simulink library "ControLibrary"  (R2015b)
settings: Solver=ode45  SolverMode=SingleTasking  StartTime=0.0  StopTime=10.0  RelTol=1e-3
values from neighbouring files (symbols this model uses):
  ControlSampleTime = 1/8000    (= 0.000125)    [initTPHardware.m]
  DCCC = initDCCC(LCL,SM)    [Sim_TP3_VSM_init.m]    (also in initDCCC.m = initHSS(LCL,SM))
undefined symbols (not defined in the file or in its folder): CCCTRL, DiscIntNeverNeededParam, VSMCTRL
undefined symbols (not defined in the file): HSS, VSMCC
libraries: FriedrichLibrary x46, simulink x23, simulink_extras x4, ControLibrary x2, ctrl_basic x2
(part 1 of 4)
settings Model: Creator=fwelck  LastModifiedBy=fwelck
settings DataIOCC: SaveFormat=Array
settings OptimizationCC: BlockReduction=off  BooleanDataType=off
settings DebuggingCC: SaveWithParameterizedLinksMsg=none  UnderspecifiedInitializationDetection=Classic  MergeDetectMultiDrivingBlocksExec=none  SignalResolutionControl=TryResolveAllWithWarning  StrictBusMsg=Warning
settings HardwareCC: ProdBitPerPointer=32  ProdLargestAtomicFloat=None  ProdIntDivRoundTo=Undefined  ProdEndianess=Unspecified  ProdWordSize=32  ProdHWDeviceType=32-bit Generic  TargetUnknown=on
settings GRTTargetCC: GeneratePreprocessorConditionals=Disable all
settings ConfigComp: CovModelRefEnable=Off  CovSFcnEnable=off

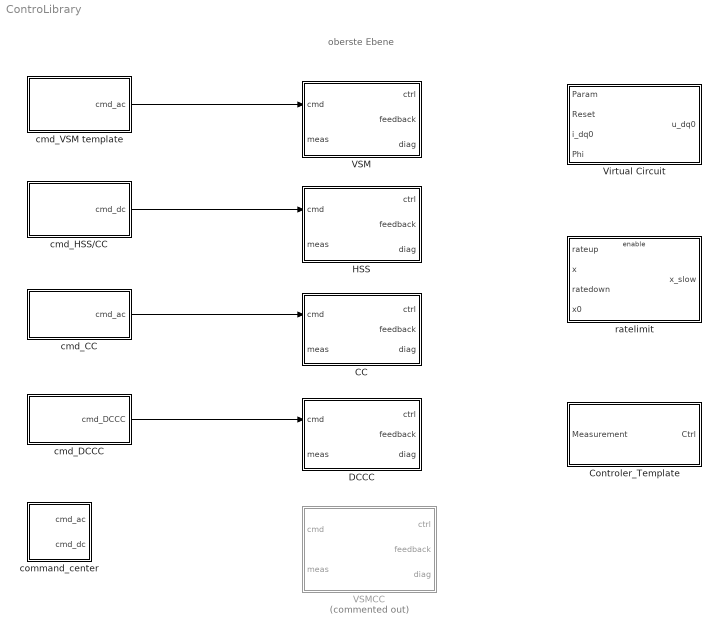
== system ControLibrary ==
  note: oberste Ebene
  CC : Subsystem  InitFcn=createTriphaseBus  mask{Ctrl=CCCTRL, pu=CCCTRL.PU, DoN=off}
      mask prompts: Ctrl "Param Struct"; pu "PU-System"; DoN "N Leiter Schalten (4 Phasen)"
      mask init:
      | if DoN
      |     NrChannels=4;
      | else
      |     NrChannels=3;
      | end
  Controler_Template : Subsystem
  DCCC : Subsystem  InitFcn=createTriphaseBus  mask{Ctrl=DCCC, PU=DCCC.PU}
      mask prompts: Ctrl "ParamStruct"; PU "PU-System"
      mask init:
      | NrChannels = 3;
  HSS : Subsystem  InitFcn=createTriphaseBus  mask{Ctrl=HSS, PU=VSMCTRL.PU}
      mask prompts: Ctrl "ParamStruct"; PU "PU-System"
  VSM : Subsystem  ClipboardFcn=createTriphaseBus  mask{Ctrl=VSMCTRL, pu=VSMCTRL.PU, DoN=off}
      mask prompts: Ctrl "ParamStruct"; pu "PU-System"; DoN "N Leiter Schalten (4 Phasen)"
      mask init:
      | if DoN
      |     NrChannels=4;
      | else
      |     NrChannels=3;
      | end
  VSMCC : Subsystem  Commented=on  mask{Ctrl=VSMCC, DoN=off}
      mask prompts: Ctrl "ParamStruct"; DoN "N Leiter Schalten (4 Phasen)"
      mask init:
      | if DoN
      |     NrChannels=4;
      | else
      |     NrChannels=3;
      | end
  Virtual Circuit : Subsystem
  cmd_CC : Subsystem
  cmd_DCCC : Subsystem
  cmd_HSS/CC : Subsystem
  cmd_VSM template : Subsystem
  command_center : Subsystem
  ratelimit : Subsystem  mask{Ts=ControlSampleTime}
      mask DialogControl ParameterGroupVar Prompt: Rate Limiter
  wires:
  cmd_VSM template/1(cmd_ac) -> VSM/1(cmd)
  cmd_HSS/CC/1(cmd_dc) -> HSS/1(cmd)
  cmd_CC/1(cmd_ac) -> CC/1(cmd)
  cmd_DCCC/1(cmd_DCCC) -> DCCC/1(cmd)

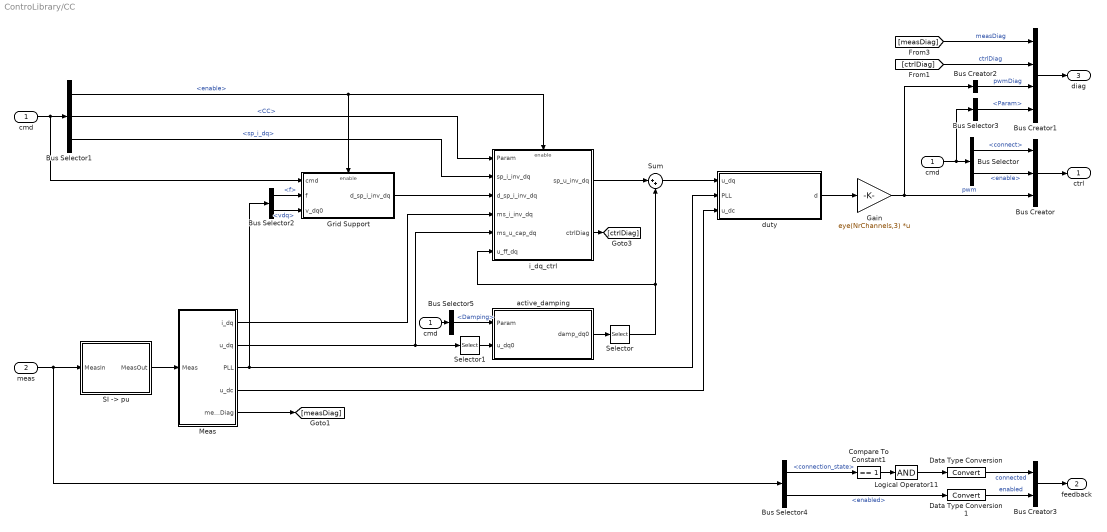
== system ControLibrary/CC ==
  cmd : Inport
  meas : Inport  Port=2
  "  cmd  " : InportShadow
  Bus Creator : BusCreator  Inputs=3
  Bus Creator1 : BusCreator  Inputs=4
  Bus Creator2 : BusCreator  Inputs=1
  Bus Selector : BusSelector  OutputSignals=Manage.connect,Manage.enable
  Bus Selector1 : BusSelector  OutputSignals=Manage.enable,Param.CC,sp_i_dq
  Bus Selector2 : BusSelector  OutputSignals=f,vdq
  Bus Selector3 : BusSelector  OutputSignals=Param
  Bus Selector4 : BusSelector  OutputSignals=connection_state,enabled
  Bus Selector5 : BusSelector  OutputSignals=Damping
  Bus Creator3 : BusCreator  Inputs=2  OutDataTypeStr=Bus: FeedbackACBus
  Compare To Constant1 : simulink/Logic and Bit Operations/Compare To Constant  relop===  const=1  OutDataTypeStr=boolean
  Data Type Conversion : DataTypeConversion
  Data Type Conversion1 : DataTypeConversion
  Gain : Gain  Gain=eye(NrChannels,3)  Multiplication=Matrix(K*u)
  Grid Support : Subsystem  mask{Omegab=pu.omegab, tauhf=1e-3}
      mask DialogControl dfdtRegler Prompt: df/dt Regler
  Logical Operator11 : Logic  Inputs=1  AllPortsSameDT=off  OutDataTypeStr=boolean
  Meas : Subsystem  mask{PLL=Ctrl.PLL}
      mask prompts: PLL "PLL Parameter"
  "SI -> pu" : Subsystem  mask{PU=pu}
      mask prompts: PU "PU System"
      mask DialogControl ParameterGroupVar Prompt: Per Unit
  Selector : Selector  InputPortWidth=3  IndexOptions=Index vector (dialog)  Indices=[1 2]  OutputSizes=1
  Selector1 : Selector  InputPortWidth=2  IndexOptions=Index vector (dialog)  Indices=[1 2 2]  OutputSizes=1
  Sum : Sum  Inputs=|++
  active_damping : Subsystem
  "cmd " : InportShadow
  duty : Subsystem
  i_dq_ctrl : Subsystem
  ctrl : Outport
  feedback : Outport  Port=2
  diag : Outport  Port=3
  wires:
  Selector1/1 -> active_damping/2(u_dq0)
  Selector/1 -> Sum/2, i_dq_ctrl/6(u_ff_dq)
  Bus Selector5/1 -> active_damping/1(Param)  "<Damping>"
  "  cmd  "/1 -> Bus Selector5/1
  Sum/1 -> duty/1(u_dq)
  i_dq_ctrl/1(sp_u_inv_dq) -> Sum/1
  Bus Selector1/2 -> i_dq_ctrl/1(Param)  "<CC>"
  Logical Operator11/1 -> Data Type Conversion/1
  Bus Selector4/1 -> Compare To Constant1/1  "<connection_state>"
  Compare To Constant1/1 -> Logical Operator11/1
  Bus Selector4/2 -> Data Type Conversion1/1  "<enabled>"
  Data Type Conversion1/1 -> Bus Creator3/2  "enabled"
  Bus Creator3/1 -> feedback/1
  Data Type Conversion/1 -> Bus Creator3/1  "connected"
  Bus Creator2/1 -> Bus Creator1/3  "pwmDiag"
  Bus Selector3/1 -> Bus Creator1/4  "<Param>"
  cmd/1 -> Bus Selector/1, Bus Selector3/1
  Grid Support/1(d_sp_i_inv_dq) -> i_dq_ctrl/3(d_sp_i_inv_dq)
  Bus Selector1/3 -> i_dq_ctrl/2(sp_i_inv_dq)  "<sp_i_dq>"
  Bus Selector1/1 -> Grid Support/Enable, i_dq_ctrl/Enable  "<enable>"
  "cmd "/1 -> Grid Support/1(cmd), Bus Selector1/1
  Bus Selector2/1 -> Grid Support/2(f)  "<f>"
  active_damping/1(damp_dq0) -> Selector/1
  Bus Creator1/1 -> diag/1
  [ctrlDiag] -> Bus Creator1/2  "ctrlDiag"
  [measDiag] -> Bus Creator1/1  "measDiag"
  Meas/5(measDiag) -> [measDiag]
  i_dq_ctrl/2(ctrlDiag) -> [ctrlDiag]
  duty/1(d) -> Gain/1
  Meas/4(u_dc) -> duty/3(u_dc)
  Meas/3(PLL) -> duty/2(PLL), Bus Selector2/1
  Meas/2(u_dq) -> i_dq_ctrl/5(ms_u_cap_dq), Selector1/1
  Gain/1 -> Bus Creator/3, Bus Creator2/1  "pwm"
  Meas/1(i_dq) -> i_dq_ctrl/4(ms_i_inv_dq)
  Bus Selector/2 -> Bus Creator/2  "<enable>"
  Bus Creator/1 -> ctrl/1
  Bus Selector/1 -> Bus Creator/1  "<connect>"
  meas/1 -> Bus Selector4/1, "SI -> pu"/1(MeasIn)
  "SI -> pu"/1(MeasOut) -> Meas/1(Meas)
  Bus Selector2/2 -> Grid Support/3(v_dq0)  "<vdq>"

== system ControLibrary/Controler_Template ==
  Measurement : Inport
  Bus Creator : BusCreator  Inputs=3
  Bus Selector : BusSelector  OutputSignals=Inv1,Inv2
  Constant : Constant  Value=0
  Constant1 : Constant  Value=0
  INV1_ctrl : Subsystem
  INV2_ctrl : Subsystem
  preload : Step  Time=0.1  SampleTime=0
  Ctrl : Outport
  wires:
  Bus Selector/2 -> INV2_ctrl/2(meas)  "<Inv2>"
  Bus Selector/1 -> INV1_ctrl/2(meas)  "<Inv1>"
  Measurement/1 -> Bus Selector/1
  preload/1 -> Bus Creator/1  "preload"
  Bus Creator/1 -> Ctrl/1
  INV2_ctrl/1(ctrl) -> Bus Creator/3  "Inv2"
  INV1_ctrl/1(ctrl) -> Bus Creator/2  "Inv1"
  Constant1/1 -> INV1_ctrl/1(cmd)
  Constant/1 -> INV2_ctrl/1(cmd)

== system ControLibrary/DCCC ==
  cmd : Inport
  meas : Inport  Port=2
  BUS_GENERATION : Subsystem
  CONTROL : Subsystem
  MANAGEMENT : Subsystem  mask{UDCbusSpMax=Ctrl.Mgn.UDCbusSpMax, UDCbusSpMin=Ctrl.Mgn.UDCbusSpMin, UDCbusSpRateUp=Ctrl.Mgn.UDCbusSpRateUp, UDCbusSpRateDown=Ctrl.Mgn.UDCbusSpRateDown, PU=PU}
      mask prompts: UDCbusSpMax "UDCbusSpMax [V]"; UDCbusSpMin "UDCbusSpMin [V]"; UDCbusSpRateUp "UDCbusSpRateUp [V/s]"; UDCbusSpRateDown "UDCbusSpRateDown [V/s]"; PU "PU-System"
      mask DialogControl GrpHssMgn Prompt: HSS Management
  Meas : Subsystem  mask(Messeinrichtung für VSM mit CC){PU=PU, PLL=Ctrl.PLL}
      mask prompts: PU "PU System"; PLL "PLL Parameters"
      mask help:
      | PU System(.Vb, .Ib)
      |
      | PLL Parameter (.kp, .ki)
      |
      | Parameter nicht auf der Maske:
      | NrChannels
      | ControlSampleTime
  ctrl : Outport  LockScale=on
  feedback : Outport  Port=2
  diag : Outport  Port=3
  wires:
  meas/1 -> Meas/1(MEASIN)
  Meas/1(MEAS) -> MANAGEMENT/2(MEAS), CONTROL/2(MEAS)
  cmd/1 -> MANAGEMENT/1(CMD)
  MANAGEMENT/1(MANAGE) -> CONTROL/1(MANAGE), BUS_GENERATION/1(MANAGE)
  CONTROL/2(diagCtrl) -> diag/1
  CONTROL/1(CONTROL) -> BUS_GENERATION/2(CONTROL)
  BUS_GENERATION/1(ctrl) -> ctrl/1
  BUS_GENERATION/2(feedback) -> feedback/1

== system ControLibrary/HSS ==
  cmd : Inport
  meas : Inport  Port=2
  BUS_GENERATION : Subsystem
  CONTROL : Subsystem
  MANAGEMENT : Subsystem  mask{UDCbusSpMax=Ctrl.Mgn.UDCbusSpMax, UDCbusSpMin=Ctrl.Mgn.UDCbusSpMin, UDCbusSpRateUp=Ctrl.Mgn.UDCbusSpRateUp, UDCbusSpRateDown=Ctrl.Mgn.UDCbusSpRateDown, PU=PU}
      mask prompts: UDCbusSpMax "UDCbusSpMax [V]"; UDCbusSpMin "UDCbusSpMin [V]"; UDCbusSpRateUp "UDCbusSpRateUp [V/s]"; UDCbusSpRateDown "UDCbusSpRateDown [V/s]"; PU "PU-System"
      mask DialogControl GrpHssMgn Prompt: HSS Management
  Meas : Subsystem
  ctrl : Outport  LockScale=on
  feedback : Outport  Port=2
  diag : Outport  Port=3
  wires:
  meas/1 -> Meas/1(MEASIN)
  Meas/1(MEAS) -> CONTROL/2(MEAS), MANAGEMENT/2(MEAS)
  CONTROL/2(ctrlDiag) -> diag/1
  BUS_GENERATION/1(ctrl) -> ctrl/1
  BUS_GENERATION/2(feedback) -> feedback/1
  CONTROL/1(CONTROL) -> BUS_GENERATION/2(CONTROL)
  MANAGEMENT/1(MANAGE) -> BUS_GENERATION/1(MANAGE), CONTROL/1(MANAGE)
  cmd/1 -> MANAGEMENT/1(CMD)

== system ControLibrary/VSM ==
  cmd : Inport
  meas : Inport  Port=2
  BUS_GENERATION : Subsystem
  CONTROL : Subsystem
  MANAGEMENT : Subsystem  mask(VSMCC Management){Mgn=Ctrl.Mgn}
      mask prompts: Mgn "Mgn Parameters"
      mask help:
      | Mgn(.PQSpRateUp, .PQSpRateDown, PQSpMax, .PQSpMin)
      |
      | Parameter nicht auf der Maske:
      | ControlSampleTime
  Meas : Subsystem  mask(Messeinrichtung für VSM mit CC){PU=pu, PLL=Ctrl.PLL}
      mask prompts: PU "PU System"; PLL "PLL Parameters"
      mask help:
      | PU System(.Vb, .Ib)
      |
      | PLL Parameter (.kp, .ki)
      |
      | Parameter nicht auf der Maske:
      | NrChannels
      | ControlSampleTime
  ctrl : Outport  LockScale=on
  feedback : Outport  Port=2
  diag : Outport  Port=3
  wires:
  Meas/1(MEAS) -> MANAGEMENT/2(MEAS), CONTROL/2(MEAS)
  MANAGEMENT/1(MANAGE) -> BUS_GENERATION/1(MANAGE), CONTROL/1(MANAGE)
  CONTROL/2(diagCtrl) -> diag/1
  BUS_GENERATION/2(feedback) -> feedback/1
  BUS_GENERATION/1(ctrl) -> ctrl/1
  CONTROL/1(CONTROL) -> BUS_GENERATION/2(CONTROL), Meas/2("CONTROL ")
  cmd/1 -> MANAGEMENT/1(CMD)
  meas/1 -> Meas/1(MEASIN)

== system ControLibrary/VSMCC ==
  cmd : Inport
  meas : Inport  Port=2
  BUS_GENERATION : Subsystem
  CONTROL : Subsystem
  MANAGEMENT : Subsystem  mask(VSMCC Management){Mgn=Ctrl.Mgn}
      mask prompts: Mgn "Mgn Parameters"
      mask help:
      | Mgn(.PQSpRateUp, .PQSpRateDown, PQSpMax, .PQSpMin)
      |
      | Parameter nicht auf der Maske:
      | ControlSampleTime
  Meas : Subsystem  mask(Messeinrichtung für VSM mit CC){PU=Ctrl.pu, PLL=Ctrl.PLL}
      mask prompts: PU "PU System"; PLL "PLL Parameters"
      mask help:
      | PU System(.Vb, .Ib)
      |
      | PLL Parameter (.kp, .ki)
      |
      | Parameter nicht auf der Maske:
      | NrChannels
      | ControlSampleTime
  ctrl : Outport  LockScale=on
  feedback : Outport  Port=2
  diag : Outport  Port=3
  wires:
  meas/1 -> Meas/1(MEASIN)
  Meas/1(MEAS) -> MANAGEMENT/2(MEAS), CONTROL/2(MEAS)
  cmd/1 -> MANAGEMENT/1(CMD)
  MANAGEMENT/1(MANAGE) -> CONTROL/1(MANAGE), BUS_GENERATION/1(MANAGE)
  CONTROL/2(diagCtrl) -> diag/1
  CONTROL/1(CONTROL) -> Meas/2("CONTROL "), BUS_GENERATION/2(CONTROL)
  BUS_GENERATION/1(ctrl) -> ctrl/1
  BUS_GENERATION/2(feedback) -> feedback/1

== system ControLibrary/Virtual Circuit ==
  Param : Inport
  Reset : Inport  Port=2
  i_dq0 : Inport  Port=3
  Phi : Inport  Port=4
  Bus Selector : BusSelector  OutputSignals=R1,L1
  Bus Selector1 : BusSelector  OutputSignals=R1t,tauR,L1t,tauL
  Current Predictor : Subsystem  Commented=on
  L_Matrix : Gain  Gain=[0 -1 0;1 0 0; 0 0 0]
  L_Matrix1 : Gain  Gain=[0 -1 0;1 0 0; 0 0 0]
  PT1 : Subsystem  mask{K=1, Init=0, Ts=ControlSampleTime}
      mask prompts: K "Gain"; Init "Initial input"; Ts "Sample time"
      mask DialogControl DescTextVar Prompt: Simple discrete PT1
      mask Display:
      | text(0.5,0.5,get_param(gcb,'K'),'HorizontalAlignment','center','VerticalAlignment','Bottom')
      | text(0.5,0.5,'1 + s.tau','HorizontalAlignment','center','VerticalAlignment','Top')
      | plot([0.3 0.7],[0.5 0.5])
  PT2 : Subsystem  mask{K=1, Init=0, Ts=ControlSampleTime}
      mask prompts: K "Gain"; Init "Initial input"; Ts "Sample time"
      mask DialogControl DescTextVar Prompt: Simple discrete PT1
      mask Display:
      | text(0.5,0.5,get_param(gcb,'K'),'HorizontalAlignment','center','VerticalAlignment','Bottom')
      | text(0.5,0.5,'1 + s.tau','HorizontalAlignment','center','VerticalAlignment','Top')
      | plot([0.3 0.7],[0.5 0.5])
  "Param " : InportShadow
  Phi1 : InportShadow  Port=4
  Product : Product  Multiplication=Matrix(*)
  Product1 : Product  Multiplication=Matrix(*)
  Product2 : Product  Multiplication=Matrix(*)
  R_Matrix : Gain  Gain=[1 0 0;0 1 0; 0 0 0]
  R_Matrix1 : Gain  Gain=[1 0 0;0 1 0; 0 0 0]
  Reset1 : InportShadow  Port=2
  Sum : Sum  Inputs=++|
  Sum1 : Sum  Inputs=++|
  Sum2 : Sum  Inputs=|++
  " u_dq0" : Outport
  wires:
  Reset1/1 -> PT2/3(Reset)
  Reset/1 -> PT1/3(Reset)
  Phi1/1 -> PT2/4(Phi)
  Phi/1 -> PT1/4(Phi)
  PT1/1(Y) -> Product1/2
  Sum2/1 -> " u_dq0"/1
  Sum1/1 -> Sum2/2
  Product2/1 -> Sum1/2
  PT2/1(Y) -> Product2/2
  L_Matrix1/1 -> Product2/1
  Bus Selector1/3 -> L_Matrix1/1  "<L1t>"
  Bus Selector1/2 -> PT1/2(tau)  "<tauR>"
  Bus Selector1/4 -> PT2/2(tau)  "<tauL>"
  Bus Selector1/1 -> R_Matrix1/1  "<R1t>"
  Product1/1 -> Sum1/1
  R_Matrix1/1 -> Product1/1
  Product/1 -> Sum2/1
  "Param "/1 -> Bus Selector1/1
  Sum/1 -> Product/1
  R_Matrix/1 -> Sum/2
  L_Matrix/1 -> Sum/1
  Bus Selector/2 -> L_Matrix/1  "<L1>"
  i_dq0/1 -> Product/2, PT1/1(U), PT2/1(U)
  Bus Selector/1 -> R_Matrix/1  "<R1>"
  Param/1 -> Bus Selector/1

== system ControLibrary/cmd_CC ==
  note: Grid Support Control
  note: Proportional Control of
      | Active current IP (f)
      | Reactive current IQ (v)
      | Derivative control of
      | Active current IP (df/dt)
  Bus Creator1 : BusCreator  Inputs=3
  Bus Creator{2,4..6} (4 alike) : BusCreator  Inputs=2
  Bus Creator3 : BusCreator  Inputs=4
  Bus Creator15 : BusCreator  Inputs=7
  Constant : Constant  Value=0
  Constant1 : Constant  Value=0
  Constant2 : Constant  Value=0
  Damping : Subsystem
  Enable Frequency Control : ManualSwitch  CurrentSetting=0
  Enable Frequency Control1 : ManualSwitch
  Enable Voltage Control : ManualSwitch
  Tai1 : Constant  Value=CCCTRL.CC.ki
  Tai2 : Constant  Value=CCCTRL.CC.xff
  Tai3 : Constant  Value=CCCTRL.IPF.k
  Tai4 : Constant  Value=CCCTRL.IQU.k
  Tai5 : Constant  Value=CCCTRL.IPF.T
  Tai6 : Constant  Value=CCCTRL.IQU.T
  Tai7 : Constant  Value=CCCTRL.CC.kp
  Tai8 : Constant  Value=CCCTRL.DFDT.Tai
  connect_ac : Constant  Value=0
  enable_ac : Constant  Value=0
  i_lim_ac : Constant  Value=25
  sp_f : Constant
  sp_i_dq : Constant  Value=[0 0]
  sp_v : Constant
  tauRi1 : Constant  Value=CCCTRL.DFDT.tauRI
  cmd_ac : Outport
  wires:
  Tai2/1 -> Bus Creator1/3  "xff"
  Damping/1(Damping) -> Bus Creator15/7  "Damping"
  Tai8/1 -> Enable Frequency Control1/1
  Constant2/1 -> Enable Frequency Control1/2
  Bus Creator4/1 -> Bus Creator15/1  "Manage"
  Tai7/1 -> Bus Creator1/2  "kp"
  Tai1/1 -> Bus Creator1/1  "ki"
  Bus Creator1/1 -> Bus Creator3/4  "CC"
  Bus Creator3/1 -> Bus Creator15/6  "Param"
  Enable Voltage Control/1 -> Bus Creator6/1  "k"
  Constant1/1 -> Enable Voltage Control/2
  Enable Frequency Control/1 -> Bus Creator5/1  "k"
  Constant/1 -> Enable Frequency Control/2
  sp_f/1 -> Bus Creator15/4  "sp_f"
  sp_v/1 -> Bus Creator15/5  "sp_v"
  Tai6/1 -> Bus Creator6/2  "T"
  Tai5/1 -> Bus Creator5/2  "T"
  Tai4/1 -> Enable Voltage Control/1  "k"
  Tai3/1 -> Enable Frequency Control/1  "k"
  Bus Creator5/1 -> Bus Creator3/2  "iP-f"
  Bus Creator6/1 -> Bus Creator3/3  "iQ-u"
  tauRi1/1 -> Bus Creator2/1  "tauRi"
  Bus Creator2/1 -> Bus Creator3/1  "dfdt"
  Enable Frequency Control1/1 -> Bus Creator2/2  "Tai"
  Bus Creator15/1 -> cmd_ac/1
  i_lim_ac/1 -> Bus Creator15/2  "i_lim"
  connect_ac/1 -> Bus Creator4/1  "connect"
  enable_ac/1 -> Bus Creator4/2  "enable"
  sp_i_dq/1 -> Bus Creator15/3  "sp_i_dq"

== system ControLibrary/cmd_DCCC ==
  Bus Creator1 : BusCreator  Inputs=3
  Bus Creator15 : BusCreator  Inputs=2
  CC Parameter : Subsystem
  Damping : Subsystem
  Manage : Subsystem
  VDC Parameter : Subsystem
  cmd_DCCC : Outport
  wires:
  Damping/1(Damping) -> Bus Creator1/3  "Damping"
  Bus Creator15/1 -> cmd_DCCC/1
  VDC Parameter/1(VDC Param) -> Bus Creator1/2  "VDC"
  Manage/1(Manage) -> Bus Creator15/1  "Manage"
  CC Parameter/1(CC) -> Bus Creator1/1  "CC"
  Bus Creator1/1 -> Bus Creator15/2  "Param"

== system ControLibrary/cmd_HSS//CC ==
  Bus Creator : BusCreator  Inputs=3
  connect : Constant
  enable : Constant
  sp_DCbus [V] : Constant  Value=720
  cmd_dc : Outport
  wires:
  Bus Creator/1 -> cmd_dc/1
  connect/1 -> Bus Creator/1  "connect"
  enable/1 -> Bus Creator/2  "enable"
  sp_DCbus [V]/1 -> Bus Creator/3  "sp_DCbus_U"

== system ControLibrary/cmd_VSM template ==
  note: Parameter
  Bus Creator1 : BusCreator  Inputs=4
  Bus Creator2 : BusCreator  Inputs=2
  Current Control : Subsystem
  Damping : Subsystem
  Manage : Subsystem
  Virtual Circuit : Subsystem
  Virtual Synchronous Machine : Subsystem
  cmd_ac : Outport
  wires:
  Bus Creator1/1 -> Bus Creator2/2  "Param"
  Manage/1(Manage) -> Bus Creator2/1  "Manage"
  Virtual Circuit/1(Virtual Circuit) -> Bus Creator1/4  "VC"
  Damping/1(Damping) -> Bus Creator1/3  "Damping"
  Current Control/1(Current Control) -> Bus Creator1/2  "CC"
  Virtual Synchronous Machine/1(Virtual Synchronous Machine) -> Bus Creator1/1  "VSM"
  Bus Creator2/1 -> cmd_ac/1

== system ControLibrary/command_center ==
  note: Per Unit!
  Bus Creator12 : BusCreator  Inputs=4
  Bus Creator15 : BusCreator  Inputs=6
  Mux : Mux  Inputs=2
  Sum : Sum  Inputs=|++
  connect_ac : Step  Time=0.4  SampleTime=0
  connect_dc : Step  Time=0.05  SampleTime=0
  enable_ac : Step  Time=0.5  SampleTime=0
  enable_dc : Step  Time=0.1  SampleTime=0
  i_lim_ac : Constant  Value=25
  id_ref : Step  Time=0.7  After=0.25  SampleTime=0
  id_ref1 : Step  After=-0.5  SampleTime=0
  iqsp : Constant  Value=0
  p_q_ac : Constant  Value=[-1 1] * 40000
  preload : Step  Time=0  SampleTime=0
  sp_current : Constant  Value=[-1, -1]*10
  sp_dcbus : Step  Time=0  Before=700  After=700  SampleTime=0
  cmd_ac : Outport
  cmd_dc : Outport  Port=2
  wires:
  sp_current/1 -> Bus Creator12/3  "sp_cs"
  sp_dcbus/1 -> Bus Creator12/4  "sp_DCbus_U"
  Bus Creator12/1 -> cmd_dc/1
  connect_dc/1 -> Bus Creator12/1  "connect"
  enable_dc/1 -> Bus Creator12/2  "enable_control"
  Bus Creator15/1 -> cmd_ac/1
  p_q_ac/1 -> Bus Creator15/5  "p_ph"
  i_lim_ac/1 -> Bus Creator15/4  "i_lim"
  connect_ac/1 -> Bus Creator15/2  "connect"
  enable_ac/1 -> Bus Creator15/3  "enable"
  preload/1 -> Bus Creator15/1  "preload"
  Mux/1 -> Bus Creator15/6  "sp_i_dq"
  id_ref/1 -> Sum/2  "id_ref"
  id_ref1/1 -> Sum/1
  Sum/1 -> Mux/1
  iqsp/1 -> Mux/2

== system ControLibrary/ratelimit ==
  rateup : Inport
  x : Inport  Port=2
  ratedown : Inport  Port=3
  x0 : Inport  Port=4
  Enable : EnablePort
  Delay : Delay  DelayLength=1  InitialConditionSource=Input port  SampleTime=Ts
      settings: InputPortMap=u0,p4
  Gain : Gain  Gain=Ts
  Gain1 : Gain  Gain=-Ts
  Saturation Dynamic2 : simulink/Discontinuities/Saturation Dynamic  OutMin=[]  OutMax=[]  OutDataTypeStr=Inherit: Same as second input  OutDataType=fixdt(1, 16)  OutScaling=2^-10  DoSatur=off
  Sum : Sum  Inputs=|+-
  Sum1 : Sum  Inputs=|++
  x_slow : Outport
  wires:
  Gain1/1 -> Saturation Dynamic2/3
  ratedown/1 -> Gain1/1
  rateup/1 -> Gain/1
  Gain/1 -> Saturation Dynamic2/1
  x0/1 -> Delay/2
  Sum1/1 -> Delay/1, x_slow/1
  Saturation Dynamic2/1 -> Sum1/1
  Sum/1 -> Saturation Dynamic2/2
  Delay/1 -> Sum/2, Sum1/2
  x/1 -> Sum/1

== system ControLibrary/CC/Grid Support ==
  cmd : Inport
  f : Inport  Port=2
  v_dq0 : Inport  Port=3
  Enable : EnablePort  StatesWhenEnabling=reset
  "  cmd  " : InportShadow
  " PT1 " : Subsystem
  " cmd " : InportShadow
  " cmd  " : InportShadow
  Abs : Abs
  Add : Sum  Inputs=-+
  Add1 : Sum  Inputs=-+|
  Add2 : Sum  Inputs=+-|
  Bus Selector6 : BusSelector  OutputSignals=sp_f
  Bus Selector7 : BusSelector  OutputSignals=sp_v
  DT1 : Subsystem
  Demux : Demux  Outputs=2
  Hz2pu : Gain  Gain=2*pi/Omegab
  Mux : Mux  Inputs=2
  PT1 tau_hf : Subsystem  mask{T=tauhf, initU0=on}
      mask prompts: T "Zeitkonstante [s]"; initU0 "Mit Startwert initialisieren"
      mask DialogControl DescGroupVar Prompt: PT1 Glied
      mask Display: dpoly(1/T,[1 1/T],'s')
  "PT1 " : Subsystem
  PT1 tau_hf : Subsystem  mask{T=tauhf, initU0=on}
      mask prompts: T "Zeitkonstante [s]"; initU0 "Mit Startwert initialisieren"
      mask DialogControl DescGroupVar Prompt: PT1 Glied
      mask Display: dpoly(1/T,[1 1/T],'s')
  Real-Imag to Complex : RealImagToComplex
  Selector : Selector  InputPortWidth=3  IndexOptions=Index vector (dialog)  Indices=[1 2]  OutputSizes=1
  T_AI tau_RI : BusSelector  OutputSignals=Param.dfdt.Tai,Param.dfdt.tauRi
  "cmd " : InportShadow
  k_Pf T_Pf : BusSelector  OutputSignals=Param.iP-f.k,Param.iP-f.T
  k_Qv T_Qv : BusSelector  OutputSignals=Param.iQ-u.k,Param.iQ-u.T
  d_sp_i_inv_dq : Outport
  wires:
  Abs/1 -> Add2/2  "v_abs"
  k_Pf T_Pf/2 -> " PT1 "/3(T)  "<T>"
  k_Pf T_Pf/1 -> " PT1 "/2(gain)  "<k>"
  PT1 tau_hf/1(y) -> DT1/1(u)
  T_AI tau_RI/1 -> DT1/2(gain)  "<Tai>"
  T_AI tau_RI/2 -> DT1/3(T)  "<tauRi>"
  k_Qv T_Qv/1 -> "PT1 "/2(gain)  "<k>"
  PT1 tau_hf/1(y) -> " PT1 "/1(u)
  f/1 -> Hz2pu/1
  Hz2pu/1 -> PT1 tau_hf/1(u), Add1/1
  Mux/1 -> d_sp_i_inv_dq/1
  cmd/1 -> T_AI tau_RI/1
  DT1/1(y) -> Add/1
  Add/1 -> Mux/1
  Add1/1 -> PT1 tau_hf/1(u)
  Bus Selector6/1 -> Add1/2  "<sp_f>"
  v_dq0/1 -> Selector/1
  Selector/1 -> Demux/1
  Demux/1 -> Real-Imag to Complex/1
  Demux/2 -> Real-Imag to Complex/2
  Real-Imag to Complex/1 -> Abs/1
  Add2/1 -> "PT1 "/1(u)
  "PT1 "/1(y) -> Mux/2
  " PT1 "/1(y) -> Add/2
  "cmd "/1 -> k_Pf T_Pf/1
  " cmd "/1 -> k_Qv T_Qv/1
  k_Qv T_Qv/2 -> "PT1 "/3(T)  "<T>"
  "  cmd  "/1 -> Bus Selector6/1
  " cmd  "/1 -> Bus Selector7/1
  Bus Selector7/1 -> Add2/1  "<sp_v>"

== system ControLibrary/CC/Meas ==
  Meas : Inport
  "3_2 " : Gain  Gain=eye(2,3)  Multiplication=Matrix(K*u)
  3_2 1 : Gain  Gain=eye(2,3)  Multiplication=Matrix(K*u)
  Bus Creator : BusCreator  Inputs=3
  Bus Creator1 : BusCreator  Inputs=2
  Bus Selector : BusSelector  OutputSignals=meas_i_inverter,meas_u_cap,meas_vol_dc
  Gain : Gain  Gain=eye(3,NrChannels)  Multiplication=Matrix(K*u)
  Gain1 : Gain  Gain=eye(3,NrChannels)  Multiplication=Matrix(K*u)
  Gain2 : Gain  Gain=2/3
  InstantPowerPhN : FriedrichLibrary/Transformations/InstantPowerPhN
  PhN->ab0 : FriedrichLibrary/Transformations/PhN->ab0  SystemSampleTime=-1
  PhN->ab2 : FriedrichLibrary/Transformations/PhN->ab0  SystemSampleTime=-1
  Symmetrical PLL : FriedrichLibrary/Discrete Stuff/Symmetrical PLL  Kp_PLL=PLL.kp  Ki_PLL=PLL.ki  Kd_PLL=0  Ts=ControlSampleTime
  ab0->dq0-faster : FriedrichLibrary/Transformations/ab0->dq0-faster  SystemSampleTime=-1
  ab0->dq0-faster1 : FriedrichLibrary/Transformations/ab0->dq0-faster  SystemSampleTime=-1
  i_dq : Outport
  u_dq : Outport  Port=2
  PLL : Outport  Port=3
  u_dc : Outport  Port=4
  measDiag : Outport  Port=5
  wires:
  Gain2/1 -> Bus Creator1/2  "PQ"
  "3_2 "/1 -> i_dq/1
  3_2 1/1 -> u_dq/1
  Bus Creator1/1 -> measDiag/1
  Bus Creator/1 -> Bus Creator1/1, PLL/1  "PLL"
  InstantPowerPhN/1 -> Gain2/1  "PQ"
  Gain1/1 -> PhN->ab0/1, Symmetrical PLL/1, InstantPowerPhN/1
  Bus Selector/2 -> Gain1/1  "<meas_u_cap>"
  ab0->dq0-faster/1 -> "3_2 "/1
  ab0->dq0-faster1/1 -> 3_2 1/1
  PhN->ab2/1 -> ab0->dq0-faster/1
  PhN->ab0/1 -> ab0->dq0-faster1/1
  Gain/1 -> PhN->ab2/1, InstantPowerPhN/2
  Symmetrical PLL/1 -> Bus Creator/1  "vdq"
  Symmetrical PLL/3 -> Bus Creator/3  "f"
  Symmetrical PLL/2 -> Bus Creator/2, ab0->dq0-faster1/2, ab0->dq0-faster/2  "phi"
  Bus Selector/1 -> Gain/1  "<meas_i_inverter>"
  Bus Selector/3 -> u_dc/1  "<meas_vol_dc>"
  Meas/1 -> Bus Selector/1

== system ControLibrary/CC/SI -> pu ==
  MeasIn : Inport
  Bus Creator1 : BusCreator  Inputs=5
  Bus Selector : BusSelector  OutputSignals=meas_u_out,meas_i_out,meas_i_inverter,meas_u_dc,meas_u_cap
  Normalize : Gain  Gain=1/PU.Vb  OutDataTypeStr=double  RndMeth=Round
  Normalize1 : Gain  Gain=1/PU.Ib  OutDataTypeStr=double  RndMeth=Round
  Normalize2 : Gain  Gain=1/PU.Ib  OutDataTypeStr=double  RndMeth=Round
  Normalize3 : Gain  Gain=1/PU.Vb  OutDataTypeStr=double  RndMeth=Round
  Normalize4 : Gain  Gain=1/PU.Vb/2  OutDataTypeStr=double  RndMeth=Round
  MeasOut : Outport
  wires:
  Normalize3/1 -> Bus Creator1/5  "meas_u_cap"
  Bus Selector/5 -> Normalize3/1  "<meas_u_cap>"
  Bus Selector/4 -> Normalize4/1  "<meas_u_dc>"
  Bus Selector/3 -> Normalize1/1  "<meas_i_inverter>"
  Bus Selector/2 -> Normalize2/1  "<meas_i_out>"
  Bus Selector/1 -> Normalize/1  "<meas_u_out>"
  Bus Creator1/1 -> MeasOut/1
  Normalize4/1 -> Bus Creator1/4  "meas_vol_dc"
  Normalize2/1 -> Bus Creator1/2  "meas_i_out"
  Normalize1/1 -> Bus Creator1/3  "meas_i_inverter"
  Normalize/1 -> Bus Creator1/1  "meas_u_out"
  MeasIn/1 -> Bus Selector/1

== system ControLibrary/CC/active_damping ==
  Param : Inport
  u_dq0 : Inport  Port=2
  Bus Selector : BusSelector  OutputSignals=Damp_dq,Damp_dq,Damp_CM,OmLead,OmLag
  Integrator (inertia) : DiscreteIntegrator  gainval=1  InitialCondition=1  InitialConditionSetting=State (most efficient)  SampleTime=ControlSampleTime  ICPrevOutput=DiscIntNeverNeededParam  ICPrevScaledInput=DiscIntNeverNeededParam
  Mux : Mux  Inputs=3
  Product{,1..3} (4 alike) : Product
  Sum : Sum  Inputs=|+-
  Sum2 : Sum  Inputs=++|
  damp_dq0 : Outport
  wires:
  u_dq0/1 -> Product/2
  Bus Selector/5 -> Product3/2  "<OmLag>"
  Bus Selector/4 -> Product2/1  "<OmLead>"
  Product2/1 -> Sum/1
  Integrator (inertia)/1 -> Sum2/2
  Product3/1 -> Sum/2
  Sum2/1 -> Product1/2, Product3/1
  Sum/1 -> Integrator (inertia)/1
  Param/1 -> Bus Selector/1
  Bus Selector/1 -> Mux/1  "<Damp_dq>"
  Bus Selector/2 -> Mux/2  "<Damp_dq>"
  Bus Selector/3 -> Mux/3  "<Damp_CM>"
  Product/1 -> Sum2/1, Product2/2
  Mux/1 -> Product/1, Product1/1  "enable"
  Product1/1 -> damp_dq0/1

== system ControLibrary/CC/duty ==
  u_dq : Inport
  PLL : Inport  Port=2
  u_dc : Inport  Port=3
  2-3 : Gain  Gain=eye(3,2)  Multiplication=Matrix(K*u)
  Bias : Bias  Bias=1.05*Ctrl.PWM.tauT*pu.omegab
  Bus Selector2 : BusSelector  OutputSignals=phi
  Divide : Product  Inputs=*/
  Modulation : FriedrichLibrary/Transformations/Modulation  Method=Sine Modulation  Ts=ControlSampleTime
  avoid divivions by 0 : Saturate  UpperLimit=Inf  LowerLimit=1
  dq0->ab0 : FriedrichLibrary/Transformations/dq0->ab0 phi  SystemSampleTime=-1
  d : Outport
  wires:
  avoid divivions by 0/1 -> Divide/2
  Bus Selector2/1 -> Bias/1  "<phi>"
  PLL/1 -> Bus Selector2/1
  2-3/1 -> dq0->ab0/1
  Divide/1 -> Modulation/1  "ab0 norm"
  dq0->ab0/1 -> Divide/1
  Modulation/1 -> d/1
  u_dq/1 -> 2-3/1
  Bias/1 -> dq0->ab0/2
  u_dc/1 -> avoid divivions by 0/1

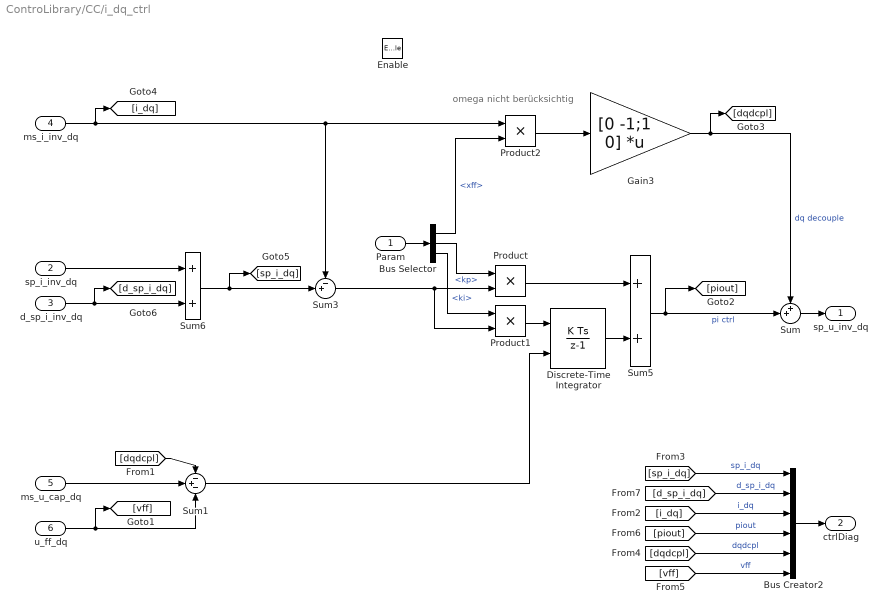
== system ControLibrary/CC/i_dq_ctrl ==
  note: omega nicht berücksichtig
  Param : Inport
  sp_i_inv_dq : Inport  Port=2
  d_sp_i_inv_dq : Inport  Port=3
  ms_i_inv_dq : Inport  Port=4
  ms_u_cap_dq : Inport  Port=5
  u_ff_dq : Inport  Port=6
  Enable : EnablePort  StatesWhenEnabling=reset
  Bus Creator2 : BusCreator  Inputs=6
  Bus Selector : BusSelector  OutputSignals=xff,kp,ki
  Discrete-Time Integrator : DiscreteIntegrator  InitialConditionSource=external  InitialConditionSetting=State (most efficient)  SampleTime=ControlSampleTime  ICPrevOutput=DiscIntNeverNeededParam  ICPrevScaledInput=DiscIntNeverNeededParam
  Gain3 : Gain  Gain=[0 -1;1 0]  Multiplication=Matrix(K*u)
  Product : Product
  Product1 : Product
  Product2 : Product
  Sum : Sum  Inputs=++|
  Sum1 : Sum  Inputs=-+-
  Sum3 : Sum  Inputs=-+|
  Sum5 : Sum
  Sum6 : Sum
  sp_u_inv_dq : Outport
  ctrlDiag : Outport  Port=2
  wires:
  Bus Selector/1 -> Product2/2  "<xff>"
  Bus Selector/3 -> Product1/1  "<ki>"
  Bus Selector/2 -> Product/1  "<kp>"
  Param/1 -> Bus Selector/1
  [d_sp_i_dq] -> Bus Creator2/2  "d_sp_i_dq"
  d_sp_i_inv_dq/1 -> Sum6/2, [d_sp_i_dq]
  Sum6/1 -> Sum3/2, [sp_i_dq]
  u_ff_dq/1 -> [vff], Sum1/3
  ms_u_cap_dq/1 -> Sum1/2
  [dqdcpl] -> Sum1/1
  Sum1/1 -> Discrete-Time Integrator/2
  Bus Creator2/1 -> ctrlDiag/1
  [sp_i_dq] -> Bus Creator2/1  "sp_i_dq"
  [i_dq] -> Bus Creator2/3  "i_dq"
  [piout] -> Bus Creator2/4  "piout"
  [vff] -> Bus Creator2/6  "vff"
  [dqdcpl] -> Bus Creator2/5  "dqdcpl"
  sp_i_inv_dq/1 -> Sum6/1
  Gain3/1 -> [dqdcpl], Sum/1  "dq decouple"
  Sum/1 -> sp_u_inv_dq/1
  Sum5/1 -> Sum/2, [piout]  "pi ctrl"
  Discrete-Time Integrator/1 -> Sum5/2
  Product/1 -> Sum5/1
  Product1/1 -> Discrete-Time Integrator/1
  Product2/1 -> Gain3/1
  ms_i_inv_dq/1 -> [i_dq], Product2/1, Sum3/1
  Sum3/1 -> Product1/2, Product/2

== system ControLibrary/Controler_Template/INV1_ctrl ==
  cmd : Inport
  meas : Inport  Port=2
  Bus Creator : BusCreator  Inputs=3
  Constant : Constant  Value=[0 0 0 0]
  Constant1 : Constant  Value=0
  Constant2 : Constant  Value=0
  Terminator : Terminator
  Terminator1 : Terminator
  ctrl : Outport
  wires:
  meas/1 -> Terminator1/1
  cmd/1 -> Terminator/1
  Constant1/1 -> Bus Creator/3  "enable"
  Bus Creator/1 -> ctrl/1
  Constant/1 -> Bus Creator/1  "pwm"
  Constant2/1 -> Bus Creator/2  "connect"

== system ControLibrary/Controler_Template/INV2_ctrl ==
  cmd : Inport
  meas : Inport  Port=2
  Bus Creator : BusCreator  Inputs=3
  Constant : Constant  Value=[0 0 0 0]
  Constant1 : Constant  Value=0
  Constant2 : Constant  Value=0
  Terminator : Terminator
  Terminator1 : Terminator
  ctrl : Outport
  wires:
  Constant2/1 -> Bus Creator/2  "connect"
  Constant/1 -> Bus Creator/1  "pwm"
  Bus Creator/1 -> ctrl/1
  Constant1/1 -> Bus Creator/3  "enable"
  cmd/1 -> Terminator/1
  meas/1 -> Terminator1/1

== system ControLibrary/DCCC/BUS_GENERATION ==
  MANAGE : Inport
  CONTROL : Inport  Port=2
  Bus Creator1 : BusCreator  Inputs=4
  Bus Selector1 : BusSelector  OutputSignals=DCBus_isset
  Bus Selector2 : BusSelector  OutputSignals=PWM
  Bus Selector3 : BusSelector  OutputSignals=ENABLED,CONNECT
  Bus Selector4 : BusSelector  OutputSignals=CONNECTED,ENABLED
  Bus Creator6 : BusCreator  Inputs=3  OutDataTypeStr=Bus: FeedbackDCBus
  Data Type Conversion{,1..4} (5 alike) : DataTypeConversion
  Signal Specification1 : SignalSpecification
  additional data1 : Constant  Value=0
  ctrl : Outport
  feedback : Outport  Port=2
  wires:
  Data Type Conversion2/1 -> Bus Creator6/3  "DCBus_isset"
  Bus Selector1/1 -> Data Type Conversion2/1  "<DCBus_isset>"
  Data Type Conversion3/1 -> Bus Creator6/1  "connected"
  Bus Selector3/2 -> Data Type Conversion1/1  "<CONNECT>"
  additional data1/1 -> Bus Creator1/4  "source_id"
  Data Type Conversion1/1 -> Bus Creator1/3  "connect"
  Data Type Conversion/1 -> Bus Creator1/2  "enable"
  Bus Selector3/1 -> Data Type Conversion/1  "<ENABLED>"
  Bus Creator6/1 -> feedback/1
  Bus Creator1/1 -> ctrl/1
  MANAGE/1 -> Bus Selector3/1, Bus Selector1/1, Bus Selector4/1
  Signal Specification1/1 -> Bus Creator1/1  "pwm"
  Data Type Conversion4/1 -> Bus Creator6/2  "enabled"
  CONTROL/1 -> Bus Selector2/1
  Bus Selector4/2 -> Data Type Conversion4/1  "<ENABLED>"
  Bus Selector4/1 -> Data Type Conversion3/1  "<CONNECTED>"
  Bus Selector2/1 -> Signal Specification1/1  "<PWM>"

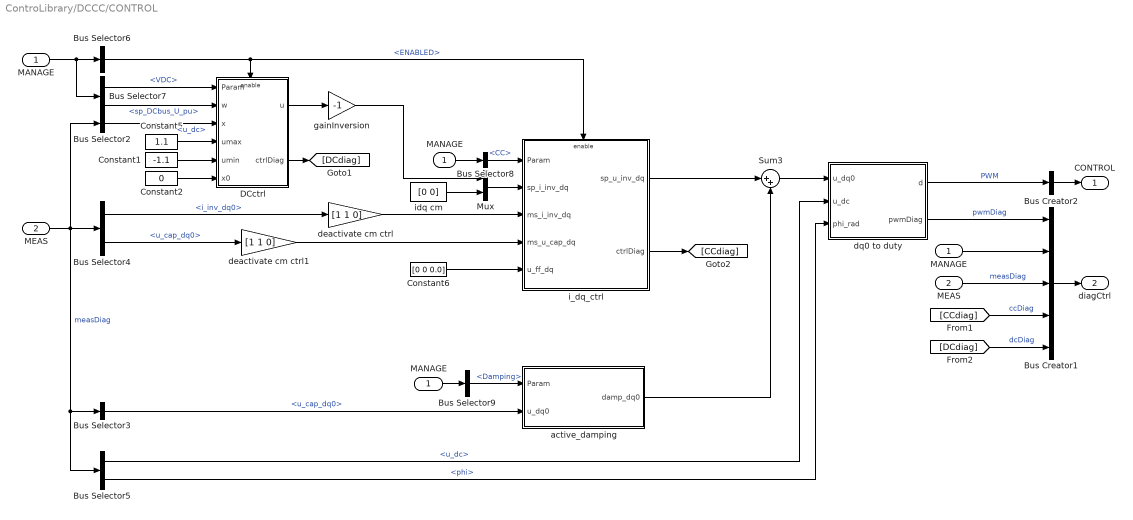
== system ControLibrary/DCCC/CONTROL ==
  MANAGE : Inport
  MEAS : Inport  Port=2
  " MANAGE" : InportShadow
  " MANAGE " : InportShadow
  Bus Creator1 : BusCreator  Inputs=5
  Bus Creator2 : BusCreator  Inputs=1
  Bus Selector2 : BusSelector  OutputSignals=u_dc
  Bus Selector3 : BusSelector  OutputSignals=u_cap.u_cap_dq0
  Bus Selector4 : BusSelector  OutputSignals=i_inv.i_inv_dq0,u_cap.u_cap_dq0
  Bus Selector5 : BusSelector  OutputSignals=u_dc,PLL.phi
  Bus Selector6 : BusSelector  OutputSignals=ENABLED
  Bus Selector7 : BusSelector  OutputSignals=Param.VDC,sp_DCbus_U_pu
  Bus Selector8 : BusSelector  OutputSignals=Param.CC
  Bus Selector9 : BusSelector  OutputSignals=Param.Damping
  Constant1 : Constant  Value=-1.1
  Constant2 : Constant  Value=0
  Constant5 : Constant  Value=1.1
  Constant6 : Constant  Value=[0 0 0.0]
  DCctrl : Subsystem
  "MANAGE " : InportShadow
  "MEAS " : InportShadow  Port=2
  Mux : Mux  Inputs=2
  Sum3 : Sum  Inputs=|++
  active_damping : Subsystem
  deactivate cm ctrl : Gain  Gain=[1 1 0]
  deactivate cm ctrl1 : Gain  Gain=[1 1 0]
  dq0 to duty : Subsystem
  gainInversion : Gain  Gain=-1
  i_dq_ctrl : Subsystem
  idq cm : Constant  Value=[0 0]
  CONTROL : Outport
  diagCtrl : Outport  Port=2
  wires:
  Bus Selector5/2 -> dq0 to duty/3(phi_rad)  "<phi>"
  deactivate cm ctrl1/1 -> i_dq_ctrl/4(ms_u_cap_dq)
  active_damping/1(damp_dq0) -> Sum3/2
  dq0 to duty/1(d) -> Bus Creator2/1  "PWM"
  deactivate cm ctrl/1 -> i_dq_ctrl/3(ms_i_inv_dq)
  i_dq_ctrl/1(sp_u_inv_dq) -> Sum3/1
  " MANAGE "/1 -> Bus Selector8/1
  Bus Selector8/1 -> i_dq_ctrl/1(Param)  "<CC>"
  Bus Selector7/1 -> DCctrl/1(Param)  "<VDC>"
  DCctrl/1(u) -> gainInversion/1
  Sum3/1 -> dq0 to duty/1(u_dq0)
  Constant6/1 -> i_dq_ctrl/5(u_ff_dq)
  gainInversion/1 -> Mux/1
  Mux/1 -> i_dq_ctrl/2(sp_i_inv_dq)
  Bus Selector9/1 -> active_damping/1(Param)  "<Damping>"
  Constant2/1 -> DCctrl/6(x0)
  idq cm/1 -> Mux/2
  Bus Selector6/1 -> DCctrl/Enable, i_dq_ctrl/Enable  "<ENABLED>"
  Bus Selector7/2 -> DCctrl/2(w)  "<sp_DCbus_U_pu>"
  "MANAGE "/1 -> Bus Selector6/1, Bus Selector7/1
  Bus Selector2/1 -> DCctrl/3(x)  "<u_dc>"
  MEAS/1 -> Bus Creator1/3  "measDiag"
  dq0 to duty/2(pwmDiag) -> Bus Creator1/1  "pwmDiag"
  Bus Creator1/1 -> diagCtrl/1
  MANAGE/1 -> Bus Creator1/2
  "MEAS "/1 -> Bus Selector4/1, Bus Selector5/1, Bus Selector3/1, Bus Selector2/1  "measDiag"
  Bus Creator2/1 -> CONTROL/1
  Bus Selector4/1 -> deactivate cm ctrl/1  "<i_inv_dq0>"
  Bus Selector4/2 -> deactivate cm ctrl1/1  "<u_cap_dq0>"
  i_dq_ctrl/2(ctrlDiag) -> [CCdiag]
  [CCdiag] -> Bus Creator1/4  "ccDiag"
  Bus Selector3/1 -> active_damping/2(u_dq0)  "<u_cap_dq0>"
  Bus Selector5/1 -> dq0 to duty/2(u_dc)  "<u_dc>"
  Constant5/1 -> DCctrl/4(umax)
  Constant1/1 -> DCctrl/5(umin)
  DCctrl/2(ctrlDiag) -> [DCdiag]
  [DCdiag] -> Bus Creator1/5  "dcDiag"
  " MANAGE"/1 -> Bus Selector9/1

== system ControLibrary/DCCC/MANAGEMENT ==
  CMD : Inport
  MEAS : Inport  Port=2
  Bus Creator : BusCreator  Inputs=6
  Bus Selector1 : BusSelector  OutputSignals=Manage.sp_DCbus_U
  Bus Selector2 : BusSelector  OutputSignals=Manage.connect
  Bus Selector3 : BusSelector  OutputSignals=connection_state
  Bus Selector4 : BusSelector  OutputSignals=u_dc
  Bus Selector5 : BusSelector  OutputSignals=Manage.enable
  Bus Selector6 : BusSelector  OutputSignals=Param
  "CMD " : InportShadow
  Compare To Constant : simulink/Logic and Bit Operations/Compare To Constant  relop===  const=1  OutDataTypeStr=boolean
  Gain : Gain  Gain=1/1/PU.Ub/2
  Gain1 : Gain  Gain=PU.Ub*2
  Logical Operator3 : Logic  AllPortsSameDT=off  OutDataTypeStr=boolean
  "MEAS " : InportShadow  Port=2
  RateLimit : Subsystem
  Signal Specification : SignalSpecification  Dimensions=1
  Signal Specification1 : SignalSpecification
  Signal Specification2 : SignalSpecification
  MANAGE : Outport
  wires:
  Bus Selector6/1 -> Bus Creator/6  "<Param>"
  Signal Specification/1 -> Bus Creator/4  "sp_DCbus_U_pu"
  Gain1/1 -> RateLimit/2(ms_dcbus)
  Bus Selector1/1 -> RateLimit/1(sp_DCBus)  "<sp_DCbus_U>"
  RateLimit/1(sp_DCBus_slow) -> Gain/1
  Gain/1 -> Signal Specification/1
  RateLimit/2(DCBus_isset) -> Bus Creator/5  "DCBus_isset"
  Bus Selector4/1 -> Gain1/1  "<u_dc>"
  Bus Selector5/1 -> Logical Operator3/2  "<enable>"
  Signal Specification1/1 -> Bus Creator/1  "CONNECT"
  Bus Selector2/1 -> Signal Specification1/1  "<connect>"
  "CMD "/1 -> Bus Selector2/1
  Compare To Constant/1 -> Signal Specification2/1
  Bus Creator/1 -> MANAGE/1
  Signal Specification2/1 -> Logical Operator3/1, Bus Creator/2  "CONNECTED"
  "MEAS "/1 -> Bus Selector4/1
  Logical Operator3/1 -> Bus Creator/3, RateLimit/Enable  "ENABLED"
  MEAS/1 -> Bus Selector3/1
  Bus Selector3/1 -> Compare To Constant/1  "<connection_state>"
  CMD/1 -> Bus Selector5/1, Bus Selector1/1, Bus Selector6/1

== system ControLibrary/DCCC/Meas ==
  MEASIN : Inport
  Bus Creator : BusCreator  Inputs=4
  Bus Creator{1..3,5} (4 alike) : BusCreator  Inputs=3
  Bus Creator4 : BusCreator  Inputs=9
  Bus Selector : BusSelector  OutputSignals=meas_i_inverter,meas_i_out,meas_u_cap,meas_u_out,meas_vol_dc
  Bus Selector1 : BusSelector  OutputSignals=connection_state,enabled
  Gain{,1..3} (4 alike) : Gain  Gain=eye(3,NrChannels)  Multiplication=Matrix(K*u)
  InstantPowerPhN : FriedrichLibrary/Transformations/InstantPowerPhN
  "SI -> pu" : Subsystem  mask{PU=PU}
      mask prompts: PU "PU System"
      mask DialogControl ParameterGroupVar Prompt: Per Unit
  Signal Specification : SignalSpecification  Dimensions=1
  Signal Specification1 : SignalSpecification  Dimensions=1
  Signal Specification2 : SignalSpecification  Dimensions=3
  Signal Specification3 : SignalSpecification  Dimensions=1
  Symmetrical PLL : FriedrichLibrary/Discrete Stuff/Symmetrical PLL  Kp_PLL=PLL.kp  Ki_PLL=PLL.ki  Kd_PLL=0  Ts=ControlSampleTime
  f-omega : Gain  Gain=2*pi
  meas_i_inv : Subsystem
  meas_i_out : Subsystem
  meas_u_cap : Subsystem
  meas_u_out : Subsystem
  MEAS : Outport
  wires:
  Gain3/1 -> meas_u_out/1(abc)
  Bus Creator5/1 -> Bus Creator4/6  "u_out"
  meas_u_out/3(dq0) -> Bus Creator5/3  "u_out_dq0"
  meas_u_out/2(ab0) -> Bus Creator5/2  "u_out_ab0"
  meas_u_out/1("abc ") -> Bus Creator5/1  "u_out_abc"
  Bus Selector/4 -> Gain3/1  "<meas_u_out>"
  Bus Creator/1 -> Bus Creator4/7  "PLL"
  Bus Selector/2 -> Gain2/1  "<meas_i_out>"
  Gain2/1 -> meas_i_out/1(abc)
  Bus Creator3/1 -> Bus Creator4/5  "u_cap"
  meas_u_cap/3(dq0) -> Bus Creator3/3  "u_cap_dq0"
  meas_u_cap/2(ab0) -> Bus Creator3/2  "u_cap_ab0"
  meas_u_cap/1("abc ") -> Bus Creator3/1  "u_cap_abc"
  Bus Creator2/1 -> Bus Creator4/4  "i_out"
  meas_i_out/3(dq0) -> Bus Creator2/3  "i_out_dq0"
  meas_i_out/2(ab0) -> Bus Creator2/2  "i_out_ab0"
  meas_i_out/1("abc ") -> Bus Creator2/1  "i_out_abc"
  Bus Creator1/1 -> Bus Creator4/3  "i_inv"
  meas_i_inv/3(dq0) -> Bus Creator1/3  "i_inv_dq0"
  meas_i_inv/2(ab0) -> Bus Creator1/2  "i_inv_ab0"
  meas_i_inv/1("abc ") -> Bus Creator1/1  "i_inv_abc"
  InstantPowerPhN/1 -> Bus Creator4/8  "PQ"
  Gain1/1 -> InstantPowerPhN/1, Symmetrical PLL/1, meas_u_cap/1(abc)
  Bus Selector/3 -> Gain1/1  "<meas_u_cap>"
  Gain/1 -> InstantPowerPhN/2, meas_i_inv/1(abc)
  Symmetrical PLL/1 -> Signal Specification2/1  "vdq"
  Symmetrical PLL/3 -> Signal Specification/1  "f"
  Symmetrical PLL/2 -> Signal Specification1/1  "phi"
  Bus Selector/1 -> Gain/1  "<meas_i_inverter>"
  Bus Selector/5 -> Signal Specification3/1  "<meas_vol_dc>"
  MEASIN/1 -> Bus Selector1/1, "SI -> pu"/1(MeasIn)
  Signal Specification/1 -> f-omega/1, Bus Creator/3  "f"
  Signal Specification1/1 -> Bus Creator/2, [phi_PLL]  "phi"
  Signal Specification2/1 -> Bus Creator/1  "vdq"
  f-omega/1 -> Bus Creator/4  "omega"
  "SI -> pu"/1(MeasOut) -> Bus Selector/1
  Signal Specification3/1 -> Bus Creator4/9  "u_dc"
  Bus Creator4/1 -> MEAS/1
  Bus Selector1/1 -> Bus Creator4/1  "<connection_state>"
  Bus Selector1/2 -> Bus Creator4/2  "<enabled>"
  [phi_PLL] -> meas_i_inv/2(phi), meas_i_out/2(phi), meas_u_cap/2(phi), meas_u_out/2(phi)

== system ControLibrary/HSS/BUS_GENERATION ==
  MANAGE : Inport
  CONTROL : Inport  Port=2
  Bus Creator1 : BusCreator  Inputs=4
  Bus Selector1 : BusSelector  OutputSignals=DCBus_isset
  Bus Selector2 : BusSelector  OutputSignals=PWM
  Bus Selector3 : BusSelector  OutputSignals=ENABLED,CONNECT
  Bus Selector4 : BusSelector  OutputSignals=CONNECTED,ENABLED
  Bus Creator6 : BusCreator  Inputs=3  OutDataTypeStr=Bus: FeedbackDCBus
  Data Type Conversion{,1..4} (5 alike) : DataTypeConversion
  Signal Specification1 : SignalSpecification
  additional data1 : Constant  Value=0
  ctrl : Outport
  feedback : Outport  Port=2
  wires:
  Data Type Conversion2/1 -> Bus Creator6/3  "DCBus_isset"
  Bus Selector1/1 -> Data Type Conversion2/1  "<DCBus_isset>"
  Data Type Conversion3/1 -> Bus Creator6/1  "connected"
  Bus Selector3/2 -> Data Type Conversion1/1  "<CONNECT>"
  additional data1/1 -> Bus Creator1/4  "source_id"
  Data Type Conversion1/1 -> Bus Creator1/3  "connect"
  Data Type Conversion/1 -> Bus Creator1/2  "enable"
  Bus Selector3/1 -> Data Type Conversion/1  "<ENABLED>"
  Bus Creator6/1 -> feedback/1
  Bus Creator1/1 -> ctrl/1
  MANAGE/1 -> Bus Selector3/1, Bus Selector1/1, Bus Selector4/1
  Signal Specification1/1 -> Bus Creator1/1  "pwm"
  Data Type Conversion4/1 -> Bus Creator6/2  "enabled"
  CONTROL/1 -> Bus Selector2/1
  Bus Selector4/2 -> Data Type Conversion4/1  "<ENABLED>"
  Bus Selector4/1 -> Data Type Conversion3/1  "<CONNECTED>"
  Bus Selector2/1 -> Signal Specification1/1  "<PWM>"

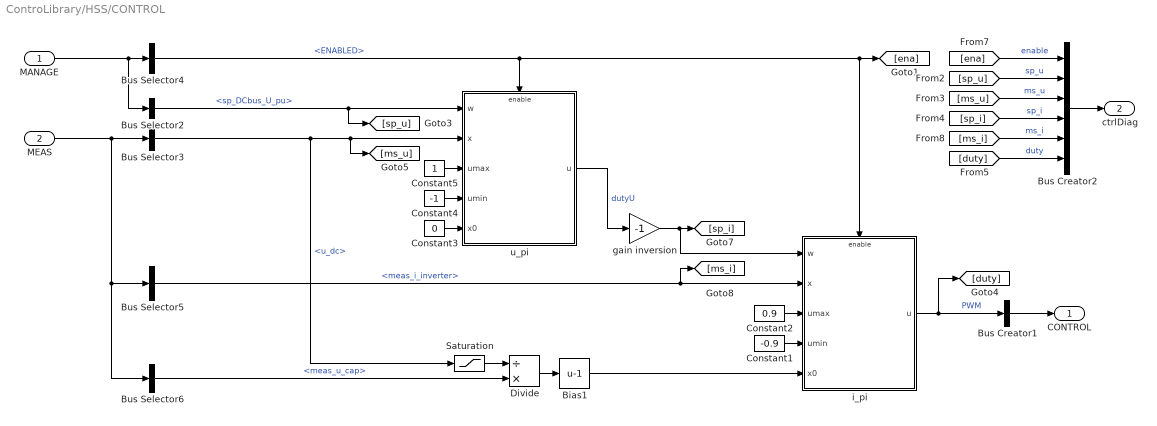
== system ControLibrary/HSS/CONTROL ==
  MANAGE : Inport
  MEAS : Inport  Port=2
  Bias1 : Bias  Bias=-1
  Bus Creator1 : BusCreator  Inputs=1
  Bus Creator2 : BusCreator  Inputs=6
  Bus Selector2 : BusSelector  OutputSignals=sp_DCbus_U_pu
  Bus Selector3 : BusSelector  OutputSignals=u_dc
  Bus Selector4 : BusSelector  OutputSignals=ENABLED
  Bus Selector5 : BusSelector  OutputSignals=meas_i_inverter
  Bus Selector6 : BusSelector  OutputSignals=meas_u_cap
  Constant1 : Constant  Value=-0.9  SampleTime=ControlSampleTime
  Constant2 : Constant  Value=0.9  SampleTime=ControlSampleTime
  Constant3 : Constant  Value=0
  Constant4 : Constant  Value=-1
  Constant5 : Constant
  Divide : Product  Inputs=/*
  Saturation : Saturate  UpperLimit=inf  LowerLimit=0.01
  gain inversion : Gain  Gain=-1
  i_pi : Subsystem  mask{kp=Ctrl.CC.kp, ki=Ctrl.CC.ki}
      mask prompts: kp "P"; ki "I"
      mask DialogControl ParameterGroupVar Prompt: PI Regler
  u_pi : Subsystem  mask{kp=Ctrl.VDC.kp, ki=Ctrl.VDC.ki}
      mask prompts: kp "P"; ki "I"
      mask DialogControl ParameterGroupVar Prompt: PI Regler
  CONTROL : Outport
  ctrlDiag : Outport  Port=2
  wires:
  Bias1/1 -> i_pi/5(x0)
  Divide/1 -> Bias1/1
  gain inversion/1 -> [sp_i], i_pi/1(w)
  Constant5/1 -> u_pi/3(umax)
  Bus Selector5/1 -> i_pi/2(x), [ms_i]  "<meas_i_inverter>"
  i_pi/1(u) -> [duty], Bus Creator1/1  "PWM"
  Bus Selector2/1 -> [sp_u], u_pi/1(w)  "<sp_DCbus_U_pu>"
  Bus Selector3/1 -> u_pi/2(x), [ms_u], Saturation/1  "<u_dc>"
  Bus Creator1/1 -> CONTROL/1
  MANAGE/1 -> Bus Selector2/1, Bus Selector4/1
  [duty] -> Bus Creator2/6  "duty"
  [ms_i] -> Bus Creator2/5  "ms_i"
  [sp_i] -> Bus Creator2/4  "sp_i"
  [ms_u] -> Bus Creator2/3  "ms_u"
  [sp_u] -> Bus Creator2/2  "sp_u"
  Bus Creator2/1 -> ctrlDiag/1
  u_pi/1(u) -> gain inversion/1  "dutyU"
  [ena] -> Bus Creator2/1  "enable"
  Constant2/1 -> i_pi/3(umax)
  Constant1/1 -> i_pi/4(umin)
  Constant4/1 -> u_pi/4(umin)
  Constant3/1 -> u_pi/5(x0)
  Bus Selector6/1 -> Divide/2  "<meas_u_cap>"
  Saturation/1 -> Divide/1
  Bus Selector4/1 -> u_pi/Enable, i_pi/Enable, [ena]  "<ENABLED>"
  MEAS/1 -> Bus Selector5/1, Bus Selector6/1, Bus Selector3/1

== system ControLibrary/HSS/MANAGEMENT ==
  CMD : Inport
  MEAS : Inport  Port=2
  Bus Creator : BusCreator  Inputs=5
  Bus Selector1 : BusSelector  OutputSignals=sp_DCbus_U
  Bus Selector2 : BusSelector  OutputSignals=connect
  Bus Selector3 : BusSelector  OutputSignals=connection_state
  Bus Selector4 : BusSelector  OutputSignals=u_dc
  Bus Selector5 : BusSelector  OutputSignals=enable
  "CMD " : InportShadow
  Compare To Constant : simulink/Logic and Bit Operations/Compare To Constant  relop===  const=1  OutDataTypeStr=boolean
  Gain : Gain  Gain=1/1/PU.Ub/2
  Gain1 : Gain  Gain=PU.Ub*2
  Logical Operator3 : Logic  AllPortsSameDT=off  OutDataTypeStr=boolean
  Logical Operator1 : Logic  Inputs=1  AllPortsSameDT=off  OutDataTypeStr=boolean
  Logical Operator2 : Logic  Inputs=1  AllPortsSameDT=off  OutDataTypeStr=boolean
  "MEAS " : InportShadow  Port=2
  RateLimit : Subsystem
  Signal Specification1 : SignalSpecification
  Signal Specification2 : SignalSpecification
  MANAGE : Outport
  wires:
  Gain1/1 -> RateLimit/2(ms_dcbus)
  Bus Selector1/1 -> RateLimit/1(sp_DCBus)  "<sp_DCbus_U>"
  RateLimit/1(sp_DCBus_slow) -> Gain/1
  Gain/1 -> Bus Creator/4  "sp_DCbus_U_pu"
  RateLimit/2(DCBus_isset) -> Bus Creator/5  "DCBus_isset"
  Bus Selector4/1 -> Gain1/1  "<u_dc>"
  Bus Selector5/1 -> Logical Operator2/1  "<enable>"
  Logical Operator2/1 -> Logical Operator3/2
  Signal Specification1/1 -> Bus Creator/1  "CONNECT"
  Bus Selector2/1 -> Signal Specification1/1  "<connect>"
  "CMD "/1 -> Bus Selector2/1
  Compare To Constant/1 -> Logical Operator1/1
  Logical Operator1/1 -> Signal Specification2/1
  Bus Creator/1 -> MANAGE/1
  Signal Specification2/1 -> Logical Operator3/1, Bus Creator/2  "CONNECTED"
  "MEAS "/1 -> Bus Selector4/1
  Logical Operator3/1 -> Bus Creator/3, RateLimit/Enable  "ENABLED"
  MEAS/1 -> Bus Selector3/1
  Bus Selector3/1 -> Compare To Constant/1  "<connection_state>"
  CMD/1 -> Bus Selector5/1, Bus Selector1/1

== system ControLibrary/HSS/Meas ==
  MEASIN : Inport
  Bus Creator4 : BusCreator  Inputs=8
  Bus Selector : BusSelector  OutputSignals=meas_i_inverter,meas_i_out,meas_u_cap,meas_u_out,meas_vol_dc
  Bus Selector1 : BusSelector  OutputSignals=connection_state,enabled
  Gain : Gain  Gain=2/3
  Product1 : Product
  "SI -> pu" : Subsystem  mask{PU=PU}
      mask prompts: PU "PU System"
      mask DialogControl ParameterGroupVar Prompt: Per Unit
  Signal Specification3 : SignalSpecification  Dimensions=1
  Sum of Elements : Sum  Inputs=+
  MEAS : Outport
  wires:
  Sum of Elements/1 -> Gain/1
  Product1/1 -> Sum of Elements/1
  Gain/1 -> Bus Creator4/7  "PQ"
  Bus Selector1/2 -> Bus Creator4/2  "<enabled>"
  Bus Selector1/1 -> Bus Creator4/1  "<connection_state>"
  Bus Creator4/1 -> MEAS/1
  Signal Specification3/1 -> Bus Creator4/8  "u_dc"
  "SI -> pu"/1(MeasOut) -> Bus Selector/1
  MEASIN/1 -> "SI -> pu"/1(MeasIn), Bus Selector1/1
  Bus Selector/5 -> Signal Specification3/1  "<meas_vol_dc>"
  Bus Selector/1 -> Bus Creator4/3, Product1/2  "<meas_i_inverter>"
  Bus Selector/2 -> Bus Creator4/4  "<meas_i_out>"
  Bus Selector/3 -> Bus Creator4/5, Product1/1  "<meas_u_cap>"
  Bus Selector/4 -> Bus Creator4/6  "<meas_u_out>"

== system ControLibrary/VSM/BUS_GENERATION ==
  MANAGE : Inport
  CONTROL : Inport  Port=2
  Bus Creator1 : BusCreator  Inputs=4
  Bus Selector2 : BusSelector  OutputSignals=PWM
  Bus Selector3 : BusSelector  OutputSignals=ENABLED,CONNECT
  Bus Selector4 : BusSelector  OutputSignals=CONNECTED,ENABLED
  Bus Creator6 : BusCreator  Inputs=2  OutDataTypeStr=Bus: FeedbackACBus
  Data Type Conversion{,1..3} (4 alike) : DataTypeConversion
  Signal Specification1 : SignalSpecification
  additional data1 : Constant  Value=0
  ctrl : Outport
  feedback : Outport  Port=2
  wires:
  Bus Selector2/1 -> Signal Specification1/1  "<PWM>"
  Bus Selector4/1 -> Data Type Conversion3/1  "<CONNECTED>"
  Bus Selector4/2 -> Data Type Conversion2/1  "<ENABLED>"
  CONTROL/1 -> Bus Selector2/1
  Data Type Conversion2/1 -> Bus Creator6/2  "enabled"
  Signal Specification1/1 -> Bus Creator1/1  "pwm"
  MANAGE/1 -> Bus Selector3/1, Bus Selector4/1
  Bus Creator1/1 -> ctrl/1
  Bus Creator6/1 -> feedback/1
  Bus Selector3/1 -> Data Type Conversion/1  "<ENABLED>"
  Data Type Conversion/1 -> Bus Creator1/2  "enable"
  Data Type Conversion1/1 -> Bus Creator1/3  "connect"
  additional data1/1 -> Bus Creator1/4  "source_id"
  Bus Selector3/2 -> Data Type Conversion1/1  "<CONNECT>"
  Data Type Conversion3/1 -> Bus Creator6/1  "connected"
